simulink model "pada_plant_model_testing"  (R2022b)
settings: Solver=VariableStepAuto  StartTime=0.0  StopTime=20  RelTol=1e-3
values from neighbouring files (symbols this model uses):
  A_lon = [du_u,  du_w,   du_q,   du_theta ... (first row only)    [pada_linear_model.m]
  B_lon = [du_de,     du_dt ... (first row only)    [pada_linear_model.m]
  C_D0 = 0.0159    [pada_aero_coefficients.m]
  C_Dalpha = 0    [pada_aero_coefficients.m]
  C_Dde = 0    [pada_aero_coefficients.m]
  C_Dq = 0    [pada_aero_coefficients.m]
  C_l0 = 0.0033    [pada_aero_coefficients.m]
  C_L0 = 0.0193    [pada_aero_coefficients.m]
  C_Lalpha = 0.056    [pada_aero_coefficients.m]
  C_lbeta = -0.04415    [pada_aero_coefficients.m]
  C_lda = 0.0025326    [pada_aero_coefficients.m]
  C_Lde = 0    [pada_aero_coefficients.m]
  C_lon = eye(4)    [pada_linear_model.m]
  C_Lq = 3.48391    [pada_aero_coefficients.m]
  C_m0 = 0.00045    [pada_aero_coefficients.m]
  C_malpha = -0.3787    [pada_aero_coefficients.m]
  C_mde = 0    [pada_aero_coefficients.m]
  C_mq = -1.26832    [pada_aero_coefficients.m]
  C_n0 = 0    [pada_aero_coefficients.m]
  C_nbeta = 0.12637    [pada_aero_coefficients.m]
  C_nda = 0    [pada_aero_coefficients.m]
  C_Xde = C_Xde    [pada_linear_model.m]
  C_Y0 = 0    [pada_aero_coefficients.m]
  C_Ybeta = -0.6377    [pada_aero_coefficients.m]
  C_Yda = 0    [pada_aero_coefficients.m]
  C_Yp = -0.06787    [pada_aero_coefficients.m]
  C_Yr = 0.51996    [pada_aero_coefficients.m]
  C_Zde = C_Zde    [pada_linear_model.m]
  D_lon = zeros(4,2)    [pada_linear_model.m]
  g = 9.81    [pada_plant.m]
  J_x = 1    [pada_plant.m]
  J_xz = 1    [pada_plant.m]
  J_y = 1    [pada_plant.m]
  J_z = 1    [pada_plant.m]
  k_motor = 1    [pada_plant.m]
  m = 1    [pada_plant.m]
  q_0 = 0    [pada_linear_model.m]
  Ref_area = 1    [pada_plant.m]
  Ref_chord = 1    [pada_plant.m]
  Ref_span = 1    [pada_plant.m]
  rho = 1    [pada_plant.m]
  S_prop = 1    [pada_plant.m]
  theta_0 = 0.01    [pada_linear_model.m]
  u_0 = 10.0    (= 10)    [pada_linear_model.m]
  w_0 = 1.0    (= 1)    [pada_linear_model.m]
undefined symbols (not defined in the file or in its folder): C_Xda, C_Zda, K_lon
libraries: simulink_extras x5, slpidlib x4, shared6dof x3, aerolibasang x3, sharedtransform x1, uavutilslib x1
(part 1 of 2)
settings Model: Creator=zachary  LastModifiedBy=zacha

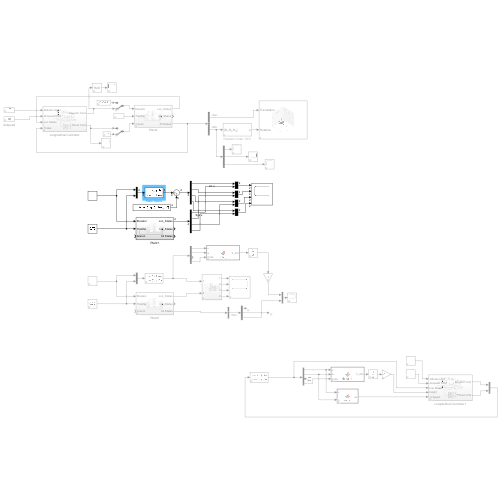
[thumbnail: Simulink's stored preview of the top-level diagram]
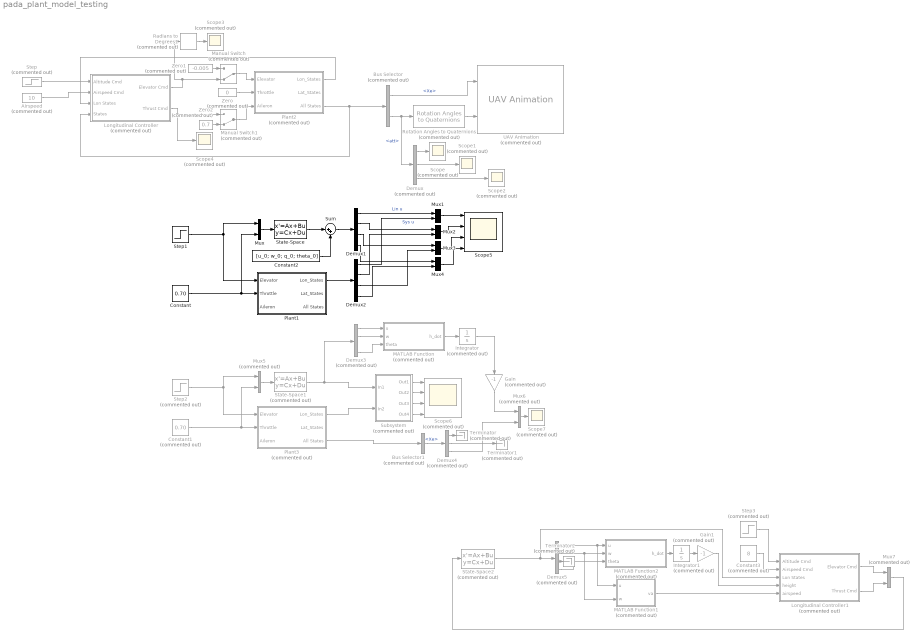
== system pada_plant_model_testing ==
  Airspeed : Constant  Commented=on  Value=10
  Bus Selector : BusSelector  Commented=on  OutputSignals=Xe,att
  Bus Selector1 : BusSelector  Commented=on  OutputSignals=Xe
  Constant : Constant  Value=0.70
  Constant1 : Constant  Commented=on  Value=0.70
  Constant2 : Constant  Value=[u_0; w_0; q_0; theta_0]
  Constant3 : Constant  Commented=on  Value=8
  Demux : Demux  Commented=on  Outputs=3
  Demux1 : Demux
  Demux2 : Demux
  Demux3 : Demux  Commented=on
  Demux4 : Demux  Commented=on  Outputs=3
  Demux5 : Demux  Commented=on
  Gain : Gain  Commented=on  Gain=-1
  Gain1 : Gain  Commented=on  Gain=-1
  Integrator : Integrator  Commented=on
  Integrator1 : Integrator  Commented=on
  Longitudinal Controller : Subsystem  Commented=on
  Longitudinal Controller1 : Subsystem  Commented=on
  MATLAB Function : MATLAB Function  Commented=on  TreatAsAtomicUnit=on
  MATLAB Function1 : MATLAB Function  Commented=on  TreatAsAtomicUnit=on
  MATLAB Function2 : MATLAB Function  Commented=on  TreatAsAtomicUnit=on
  Manual Switch : ManualSwitch  Commented=on  CurrentSetting=0
  Manual Switch1 : ManualSwitch  Commented=on  CurrentSetting=0
  Mux{,1..4} (5 alike) : Mux  Inputs=2
  Mux5 : Mux  Commented=on  Inputs=2
  Mux6 : Mux  Commented=on  Inputs=2
  Mux7 : Mux  Commented=on  Inputs=2
  Plant1 : Subsystem
  Plant2 : Subsystem  Commented=on
  Plant3 : Subsystem  Commented=on
  Radians to Degrees1 : simulink_extras/Transformations/Radians to Degrees  Commented=on
  Rotation Angles to Quaternions : sharedtransform/Rotation Angles to Quaternions  Commented=on  rotationOrder=ZYX  aMode=aMode
  Scope{,1..4,7} (6 alike) : Scope  Commented=on
  Scope5 : Scope  NumInputPorts=4
  Scope6 : Scope  Commented=on  NumInputPorts=4
  State-Space : StateSpace  A=A_lon  B=B_lon  C=C_lon  D=D_lon  InitialCondition=0
  State-Space1 : StateSpace  Commented=on  A=A_lon  B=B_lon  C=C_lon  D=D_lon  InitialCondition=0
  State-Space2 : StateSpace  Commented=on  A=A_lon  B=B_lon  C=C_lon  D=D_lon  InitialCondition=0
  Step : Step  Commented=on  After=0  SampleTime=0
  Step1 : Step  After=0.1  SampleTime=0
  Step2 : Step  Commented=on  After=0.1  SampleTime=0
  Step3 : Step  Commented=on  After=20  SampleTime=0
  Subsystem : Subsystem  Commented=on
  Sum : Sum  Inputs=|++
  Terminator : Terminator  Commented=on
  Terminator1 : Terminator  Commented=on
  Terminator2 : Terminator  Commented=on
  UAV Animation : uavutilslib/UAV Animation  Commented=on  UAVType=FixedWing  UAVSize=1  InertialZDirection=Down  SampleTime=-1
  Zero : Constant  Commented=on  Value=0  OutDataTypeStr=Inherit: Inherit via back propagation
  Zero1 : Constant  Commented=on  Value=-0.005  OutDataTypeStr=Inherit: Inherit via back propagation
  Zero2 : Constant  Commented=on  Value=0.7  OutDataTypeStr=Inherit: Inherit via back propagation
  wires:
  Plant2/3(All States) -> Bus Selector/1, Longitudinal Controller/4(States)
  Bus Selector/1 -> UAV Animation/1  "<Xe>"
  Bus Selector/2 -> Demux/1, Rotation Angles to Quaternions/1  "<att>"
  Rotation Angles to Quaternions/1 -> UAV Animation/2
  Zero/1 -> Plant2/2(Throttle)
  Zero2/1 -> Manual Switch1/2
  Zero1/1 -> Manual Switch/1
  Demux/1 -> Scope/1
  Demux/2 -> Scope1/1
  Demux/3 -> Scope2/1
  Manual Switch/1 -> Plant2/1(Elevator)
  Manual Switch1/1 -> Plant2/3(Aileron)
  Radians to Degrees1/1 -> Scope3/1
  Longitudinal Controller/1(Elevator Cmd) -> Radians to Degrees1/1, Manual Switch/2
  Longitudinal Controller/2(Thrust Cmd) -> Scope4/1, Manual Switch1/1
  Step/1 -> Longitudinal Controller/1(Altitude Cmd)
  Plant2/1(Lon_States) -> Longitudinal Controller/3(Lon States)
  Airspeed/1 -> Longitudinal Controller/2(Airspeed Cmd)
  Mux/1 -> State-Space/1
  State-Space/1 -> Sum/1
  Plant1/1(Lon_States) -> Demux2/1
  Step1/1 -> Mux/1, Plant1/1(Elevator)
  Constant/1 -> Mux/2, Plant1/2(Throttle)
  Mux1/1 -> Scope5/1
  Demux1/1 -> Mux1/1  "Lin u"
  Demux2/1 -> Mux1/2  "Sys u"
  Mux2/1 -> Scope5/2
  Mux3/1 -> Scope5/3
  Mux4/1 -> Scope5/4
  Demux1/2 -> Mux2/1
  Demux2/2 -> Mux2/2
  Demux1/3 -> Mux3/1
  Demux2/3 -> Mux3/2
  Demux1/4 -> Mux4/1
  Demux2/4 -> Mux4/2
  Constant1/1 -> Plant3/2(Throttle), Mux5/2
  Step2/1 -> Mux5/1, Plant3/1(Elevator)
  Mux5/1 -> State-Space1/1
  State-Space1/1 -> Demux3/1, Subsystem/1(In1)
  Plant3/1(Lon_States) -> Subsystem/2(In2)
  Subsystem/1(Out1) -> Scope6/1
  Subsystem/2(Out2) -> Scope6/2
  Subsystem/3(Out3) -> Scope6/3
  Subsystem/4(Out4) -> Scope6/4
  Demux3/1 -> MATLAB Function/1(u)
  Demux3/2 -> MATLAB Function/2(w)
  Demux3/4 -> MATLAB Function/3(theta)
  Plant3/3(All States) -> Bus Selector1/1
  Bus Selector1/1 -> Demux4/1  "<Xe>"
  MATLAB Function/1(h_dot) -> Integrator/1
  Mux6/1 -> Scope7/1
  Integrator/1 -> Gain/1
  Demux4/3 -> Mux6/2
  Demux4/1 -> Terminator/1
  Demux4/2 -> Terminator1/1
  Gain/1 -> Mux6/1
  Gain1/1 -> Longitudinal Controller1/4(height)
  Demux5/4 -> MATLAB Function2/3(theta)
  Demux5/2 -> MATLAB Function1/2(w), MATLAB Function2/2(w)
  State-Space2/1 -> Demux5/1, Longitudinal Controller1/3(Lon States)
  MATLAB Function2/1(h_dot) -> Integrator1/1
  Demux5/1 -> MATLAB Function1/1(u), MATLAB Function2/1(u)
  Integrator1/1 -> Gain1/1
  Demux5/3 -> Terminator2/1
  MATLAB Function1/1(va) -> Longitudinal Controller1/5(airspeed)
  Longitudinal Controller1/1(Elevator Cmd) -> Mux7/1
  Longitudinal Controller1/2(Thrust Cmd) -> Mux7/2
  Mux7/1 -> State-Space2/1
  Step3/1 -> Longitudinal Controller1/1(Altitude Cmd)
  Constant3/1 -> Longitudinal Controller1/2(Airspeed Cmd)
  Sum/1 -> Demux1/1
  Constant2/1 -> Sum/2

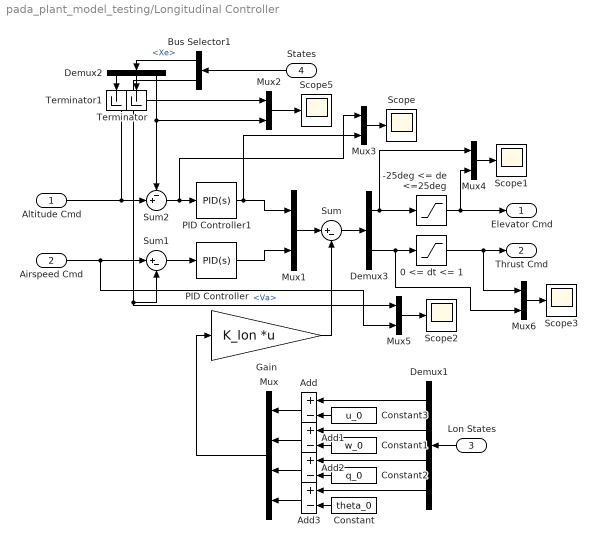
== system pada_plant_model_testing/Longitudinal Controller ==
  Altitude Cmd : Inport
  Airspeed Cmd : Inport  Port=2
  Lon States : Inport  Port=3
  States : Inport  Port=4
  -25deg <= de <=25deg : Saturate
  0 <= dt <= 1 : Saturate  UpperLimit=1  LowerLimit=0
  Add{,1..3} (4 alike) : Sum  Inputs=+-
  Bus Selector1 : BusSelector  OutputSignals=Xe,Va
  Constant : Constant  Value=theta_0  VectorParams1D=off
  Constant1 : Constant  Value=w_0  VectorParams1D=off
  Constant2 : Constant  Value=q_0  VectorParams1D=off
  Constant3 : Constant  Value=u_0  VectorParams1D=off
  Demux1 : Demux
  Demux2 : Demux  Outputs=3
  Demux3 : Demux  Outputs=2
  Gain : Gain  Gain=K_lon  Multiplication=Matrix(K*u)
  Mux : Mux
  Mux{1..6} (6 alike) : Mux  Inputs=2
  PID Controller : slpidlib/PID Controller  Controller=PID  Form=Parallel  TimeDomain=Continuous-time  UseExternalTs=off  SampleTime=-1  IntegratorMethod=Forward Euler  FilterMethod=Forward Euler  ControllerParametersSource=internal  P=0  I=0  UseKiTs=off  D=0  N=15  UseFilter=on  TunerSelectOption=Transfer Function Based (PID Tuner App)  InitialConditionSource=internal  InitialConditionForIntegrator=0  InitialConditionForFilter=0  DifferentiatorICPrevScaledInput=0  ExternalReset=none  TrackingMode=off  Kt=1  LimitOutput=off  SatLimitsSource=internal  UpperSaturationLimit=inf  LowerSaturationLimit=-inf  LinearizeAsGain=on  AntiWindupMode=none  Kb=1  LimitIntegrator=off  UpperIntegratorSaturationLimit=inf  LowerIntegratorSaturationLimit=-inf  POutMin=[]  POutMax=[]  IOutMin=[]  IOutMax=[]  DOutMin=[]  DOutMax=[]  NOutMin=[]  NOutMax=[]  SumOutMin=[]  SumOutMax=[]  SaturationOutMin=[]  SaturationOutMax=[]  PParamMin=[]  PParamMax=[]  IParamMin=[]  IParamMax=[]  DParamMin=[]  DParamMax=[]  NParamMin=[]  NParamMax=[]  KbParamMin=[]  KbParamMax=[]  KtParamMin=[]  KtParamMax=[]  KbOutMin=[]  KbOutMax=[]  KtOutMin=[]  KtOutMax=[]  IntegratorOutMin=[]  IntegratorOutMax=[]  FilterOutMin=[]  FilterOutMax=[]  SumI1OutMin=[]  SumI1OutMax=[]  SumI2OutMin=[]  SumI2OutMax=[]  SumI3OutMin=[]  SumI3OutMax=[]  SumI4OutMin=[]  SumI4OutMax=[]  SumDOutMin=[]  SumDOutMax=[]  DifferentiatorOutMin=[]  DifferentiatorOutMax=[]  FilterDiffOutCoefMin=[]  FilterDiffOutCoefMax=[]  ReciprocalOutMin=[]  ReciprocalOutMax=[]  SumDenOutMin=[]  SumDenOutMax=[]  SumNumOutMin=[]  SumNumOutMax=[]  DivideOutMin=[]  DivideOutMax=[]  UdiffTsProdOutMin=[]  UdiffTsProdOutMax=[]  NTsProdOutMin=[]  NTsProdOutMax=[]  UintegralTsProdOutMin=[]  UintegralTsProdOutMax=[]  UngainTsProdOutMin=[]  UngainTsProdOutMax=[]  ClampingZeroOutDataTypeStr=Inherit: Inherit via back propagation  ClampingZeroOutMin=[]  ClampingZeroOutMax=[]  FilterDenConstantOutDataTypeStr=Inherit: Inherit via back propagation  FilterDenConstantOutMin=[]  FilterDenConstantOutMax=[]  PCopyOutDataTypeStr=Inherit: Inherit via back propagation  PCopyOutMin=[]  PCopyOutMax=[]  NCopyOutDataTypeStr=Inherit: Inherit via back propagation  NCopyOutMin=[]  NCopyOutMax=[]  IntegratorContinuousStateAttributes=''  IntegratorStateMustResolveToSignalObject=off  IntegratorRTWStateStorageClass=Auto  FilterContinuousStateAttributes=''  FilterStateMustResolveToSignalObject=off  FilterRTWStateStorageClass=Auto  ParallelPVariant=InternalParameters  IdealPVariant=Disabled  IVariant=InternalParameters  DVariant=InternalParameters  IntegratorVariant=Continuous  SatVariant=Disabled  AWVariant=Passthrough  PCopyVariant=Disabled  TRVariant=Disabled  FdbkBlocksVariant=Forward  IdealPFdbkVariant=Disabled  SatFdbkVariant=Disabled  DerivativeFilterVariant=ContFilter  NVariant=InternalParameters  NCopyVariant=Disabled  FilterICVariant=InternalICsFilter  IntegratorICVariant=InternalICs  ExternalResetVariant=Disabled  TRSumVariant=Passthrough  SumFdbkVariant=Disabled  SumVariant=Sum_PID  TsampFilterVariant=InternalTs  TsampNgainVariant=Passthrough  TsampIntegralVariant=Passthrough  ExternalSaturationOutDataTypeStr=Inherit: Same as second input
  PID Controller1 : slpidlib/PID Controller  Controller=PID  Form=Parallel  TimeDomain=Continuous-time  UseExternalTs=off  SampleTime=-1  IntegratorMethod=Forward Euler  FilterMethod=Forward Euler  ControllerParametersSource=internal  P=1  I=0  UseKiTs=off  D=0  N=15  UseFilter=on  TunerSelectOption=Transfer Function Based (PID Tuner App)  InitialConditionSource=internal  InitialConditionForIntegrator=0  InitialConditionForFilter=0  DifferentiatorICPrevScaledInput=0  ExternalReset=none  TrackingMode=off  Kt=1  LimitOutput=off  SatLimitsSource=internal  UpperSaturationLimit=inf  LowerSaturationLimit=-inf  LinearizeAsGain=on  AntiWindupMode=none  Kb=1  LimitIntegrator=off  UpperIntegratorSaturationLimit=inf  LowerIntegratorSaturationLimit=-inf  POutMin=[]  POutMax=[]  IOutMin=[]  IOutMax=[]  DOutMin=[]  DOutMax=[]  NOutMin=[]  NOutMax=[]  SumOutMin=[]  SumOutMax=[]  SaturationOutMin=[]  SaturationOutMax=[]  PParamMin=[]  PParamMax=[]  IParamMin=[]  IParamMax=[]  DParamMin=[]  DParamMax=[]  NParamMin=[]  NParamMax=[]  KbParamMin=[]  KbParamMax=[]  KtParamMin=[]  KtParamMax=[]  KbOutMin=[]  KbOutMax=[]  KtOutMin=[]  KtOutMax=[]  IntegratorOutMin=[]  IntegratorOutMax=[]  FilterOutMin=[]  FilterOutMax=[]  SumI1OutMin=[]  SumI1OutMax=[]  SumI2OutMin=[]  SumI2OutMax=[]  SumI3OutMin=[]  SumI3OutMax=[]  SumI4OutMin=[]  SumI4OutMax=[]  SumDOutMin=[]  SumDOutMax=[]  DifferentiatorOutMin=[]  DifferentiatorOutMax=[]  FilterDiffOutCoefMin=[]  FilterDiffOutCoefMax=[]  ReciprocalOutMin=[]  ReciprocalOutMax=[]  SumDenOutMin=[]  SumDenOutMax=[]  SumNumOutMin=[]  SumNumOutMax=[]  DivideOutMin=[]  DivideOutMax=[]  UdiffTsProdOutMin=[]  UdiffTsProdOutMax=[]  NTsProdOutMin=[]  NTsProdOutMax=[]  UintegralTsProdOutMin=[]  UintegralTsProdOutMax=[]  UngainTsProdOutMin=[]  UngainTsProdOutMax=[]  ClampingZeroOutDataTypeStr=Inherit: Inherit via back propagation  ClampingZeroOutMin=[]  ClampingZeroOutMax=[]  FilterDenConstantOutDataTypeStr=Inherit: Inherit via back propagation  FilterDenConstantOutMin=[]  FilterDenConstantOutMax=[]  PCopyOutDataTypeStr=Inherit: Inherit via back propagation  PCopyOutMin=[]  PCopyOutMax=[]  NCopyOutDataTypeStr=Inherit: Inherit via back propagation  NCopyOutMin=[]  NCopyOutMax=[]  IntegratorContinuousStateAttributes=''  IntegratorStateMustResolveToSignalObject=off  IntegratorRTWStateStorageClass=Auto  FilterContinuousStateAttributes=''  FilterStateMustResolveToSignalObject=off  FilterRTWStateStorageClass=Auto  ParallelPVariant=InternalParameters  IdealPVariant=Disabled  IVariant=InternalParameters  DVariant=InternalParameters  IntegratorVariant=Continuous  SatVariant=Disabled  AWVariant=Passthrough  PCopyVariant=Disabled  TRVariant=Disabled  FdbkBlocksVariant=Forward  IdealPFdbkVariant=Disabled  SatFdbkVariant=Disabled  DerivativeFilterVariant=ContFilter  NVariant=InternalParameters  NCopyVariant=Disabled  FilterICVariant=InternalICsFilter  IntegratorICVariant=InternalICs  ExternalResetVariant=Disabled  TRSumVariant=Passthrough  SumFdbkVariant=Disabled  SumVariant=Sum_PID  TsampFilterVariant=InternalTs  TsampNgainVariant=Passthrough  TsampIntegralVariant=Passthrough  ExternalSaturationOutDataTypeStr=Inherit: Same as second input
  Scope{,1..3,5} (5 alike) : Scope
  Sum : Sum  Inputs=|+-
  Sum1 : Sum  Inputs=|+-
  Sum2 : Sum  Inputs=-+|
  Terminator : Terminator
  Terminator1 : Terminator
  Elevator Cmd : Outport
  Thrust Cmd : Outport  Port=2
  wires:
  Demux1/3 -> Add2/1
  Constant3/1 -> Add/2
  Mux1/1 -> Sum/1
  Bus Selector1/1 -> Demux2/1  "<Xe>"
  Demux1/2 -> Add1/1
  Demux3/1 -> Mux4/1, -25deg <= de <=25deg/1
  Mux/1 -> Gain/1
  PID Controller1/1 -> Mux3/2, Mux1/1
  Altitude Cmd/1 -> Mux2/1, Sum2/2
  Demux2/3 -> Sum2/1, Mux2/2
  Add3/1 -> Mux/4
  Mux2/1 -> Scope5/1
  Demux1/1 -> Add/1
  Constant/1 -> Add3/2
  States/1 -> Bus Selector1/1
  Demux3/2 -> Mux6/2, 0 <= dt <= 1/1
  Sum1/1 -> PID Controller/1
  Sum/1 -> Demux3/1
  Sum2/1 -> Mux3/1, PID Controller1/1
  PID Controller/1 -> Mux1/2
  0 <= dt <= 1/1 -> Mux6/1, Thrust Cmd/1
  Gain/1 -> Sum/2
  Add/1 -> Mux/1
  Constant1/1 -> Add1/2
  Add1/1 -> Mux/2
  -25deg <= de <=25deg/1 -> Mux4/2, Elevator Cmd/1
  Constant2/1 -> Add2/2
  Demux1/4 -> Add3/1
  Add2/1 -> Mux/3
  Bus Selector1/2 -> Mux5/1, Sum1/2  "<Va>"
  Airspeed Cmd/1 -> Mux5/2, Sum1/1
  Lon States/1 -> Demux1/1
  Demux2/2 -> Terminator/1
  Demux2/1 -> Terminator1/1
  Mux3/1 -> Scope/1
  Mux4/1 -> Scope1/1
  Mux5/1 -> Scope2/1
  Mux6/1 -> Scope3/1

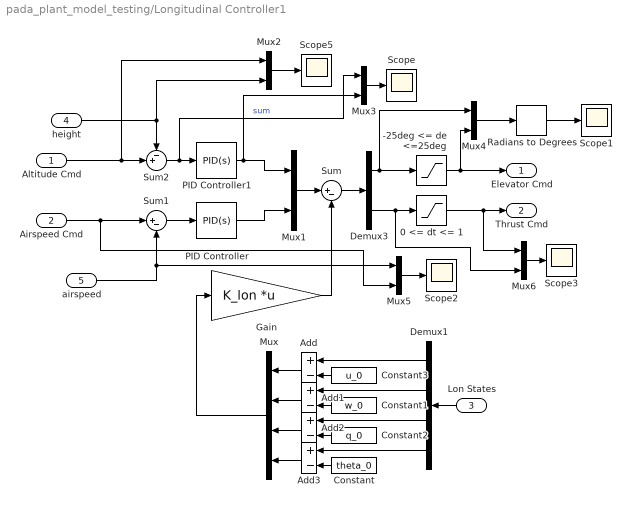
== system pada_plant_model_testing/Longitudinal Controller1 ==
  Altitude Cmd : Inport
  Airspeed Cmd : Inport  Port=2
  Lon States : Inport  Port=3
  height : Inport  Port=4
  airspeed : Inport  Port=5
  -25deg <= de <=25deg : Saturate
  0 <= dt <= 1 : Saturate  UpperLimit=1  LowerLimit=0
  Add{,1..3} (4 alike) : Sum  Inputs=+-
  Constant : Constant  Value=theta_0  VectorParams1D=off
  Constant1 : Constant  Value=w_0  VectorParams1D=off
  Constant2 : Constant  Value=q_0  VectorParams1D=off
  Constant3 : Constant  Value=u_0  VectorParams1D=off
  Demux1 : Demux
  Demux3 : Demux  Outputs=2
  Gain : Gain  Gain=K_lon  Multiplication=Matrix(K*u)
  Mux : Mux
  Mux{1..6} (6 alike) : Mux  Inputs=2
  PID Controller : slpidlib/PID Controller  Controller=PID  Form=Parallel  TimeDomain=Continuous-time  UseExternalTs=off  SampleTime=-1  IntegratorMethod=Forward Euler  FilterMethod=Forward Euler  ControllerParametersSource=internal  P=1  I=0  UseKiTs=off  D=0  N=15  UseFilter=on  TunerSelectOption=Transfer Function Based (PID Tuner App)  InitialConditionSource=internal  InitialConditionForIntegrator=0  InitialConditionForFilter=0  DifferentiatorICPrevScaledInput=0  ExternalReset=none  TrackingMode=off  Kt=1  LimitOutput=off  SatLimitsSource=internal  UpperSaturationLimit=inf  LowerSaturationLimit=-inf  LinearizeAsGain=on  AntiWindupMode=none  Kb=1  LimitIntegrator=off  UpperIntegratorSaturationLimit=inf  LowerIntegratorSaturationLimit=-inf  POutMin=[]  POutMax=[]  IOutMin=[]  IOutMax=[]  DOutMin=[]  DOutMax=[]  NOutMin=[]  NOutMax=[]  SumOutMin=[]  SumOutMax=[]  SaturationOutMin=[]  SaturationOutMax=[]  PParamMin=[]  PParamMax=[]  IParamMin=[]  IParamMax=[]  DParamMin=[]  DParamMax=[]  NParamMin=[]  NParamMax=[]  KbParamMin=[]  KbParamMax=[]  KtParamMin=[]  KtParamMax=[]  KbOutMin=[]  KbOutMax=[]  KtOutMin=[]  KtOutMax=[]  IntegratorOutMin=[]  IntegratorOutMax=[]  FilterOutMin=[]  FilterOutMax=[]  SumI1OutMin=[]  SumI1OutMax=[]  SumI2OutMin=[]  SumI2OutMax=[]  SumI3OutMin=[]  SumI3OutMax=[]  SumI4OutMin=[]  SumI4OutMax=[]  SumDOutMin=[]  SumDOutMax=[]  DifferentiatorOutMin=[]  DifferentiatorOutMax=[]  FilterDiffOutCoefMin=[]  FilterDiffOutCoefMax=[]  ReciprocalOutMin=[]  ReciprocalOutMax=[]  SumDenOutMin=[]  SumDenOutMax=[]  SumNumOutMin=[]  SumNumOutMax=[]  DivideOutMin=[]  DivideOutMax=[]  UdiffTsProdOutMin=[]  UdiffTsProdOutMax=[]  NTsProdOutMin=[]  NTsProdOutMax=[]  UintegralTsProdOutMin=[]  UintegralTsProdOutMax=[]  UngainTsProdOutMin=[]  UngainTsProdOutMax=[]  ClampingZeroOutDataTypeStr=Inherit: Inherit via back propagation  ClampingZeroOutMin=[]  ClampingZeroOutMax=[]  FilterDenConstantOutDataTypeStr=Inherit: Inherit via back propagation  FilterDenConstantOutMin=[]  FilterDenConstantOutMax=[]  PCopyOutDataTypeStr=Inherit: Inherit via back propagation  PCopyOutMin=[]  PCopyOutMax=[]  NCopyOutDataTypeStr=Inherit: Inherit via back propagation  NCopyOutMin=[]  NCopyOutMax=[]  IntegratorContinuousStateAttributes=''  IntegratorStateMustResolveToSignalObject=off  IntegratorRTWStateStorageClass=Auto  FilterContinuousStateAttributes=''  FilterStateMustResolveToSignalObject=off  FilterRTWStateStorageClass=Auto  ParallelPVariant=InternalParameters  IdealPVariant=Disabled  IVariant=InternalParameters  DVariant=InternalParameters  IntegratorVariant=Continuous  SatVariant=Disabled  AWVariant=Passthrough  PCopyVariant=Disabled  TRVariant=Disabled  FdbkBlocksVariant=Forward  IdealPFdbkVariant=Disabled  SatFdbkVariant=Disabled  DerivativeFilterVariant=ContFilter  NVariant=InternalParameters  NCopyVariant=Disabled  FilterICVariant=InternalICsFilter  IntegratorICVariant=InternalICs  ExternalResetVariant=Disabled  TRSumVariant=Passthrough  SumFdbkVariant=Disabled  SumVariant=Sum_PID  TsampFilterVariant=InternalTs  TsampNgainVariant=Passthrough  TsampIntegralVariant=Passthrough  ExternalSaturationOutDataTypeStr=Inherit: Same as second input
  PID Controller1 : slpidlib/PID Controller  Controller=PID  Form=Parallel  TimeDomain=Continuous-time  UseExternalTs=off  SampleTime=-1  IntegratorMethod=Forward Euler  FilterMethod=Forward Euler  ControllerParametersSource=internal  P=1  I=0.1  UseKiTs=off  D=0.1  N=15  UseFilter=on  TunerSelectOption=Transfer Function Based (PID Tuner App)  InitialConditionSource=internal  InitialConditionForIntegrator=0  InitialConditionForFilter=0  DifferentiatorICPrevScaledInput=0  ExternalReset=none  TrackingMode=off  Kt=1  LimitOutput=off  SatLimitsSource=internal  UpperSaturationLimit=inf  LowerSaturationLimit=-inf  LinearizeAsGain=on  AntiWindupMode=none  Kb=1  LimitIntegrator=off  UpperIntegratorSaturationLimit=inf  LowerIntegratorSaturationLimit=-inf  POutMin=[]  POutMax=[]  IOutMin=[]  IOutMax=[]  DOutMin=[]  DOutMax=[]  NOutMin=[]  NOutMax=[]  SumOutMin=[]  SumOutMax=[]  SaturationOutMin=[]  SaturationOutMax=[]  PParamMin=[]  PParamMax=[]  IParamMin=[]  IParamMax=[]  DParamMin=[]  DParamMax=[]  NParamMin=[]  NParamMax=[]  KbParamMin=[]  KbParamMax=[]  KtParamMin=[]  KtParamMax=[]  KbOutMin=[]  KbOutMax=[]  KtOutMin=[]  KtOutMax=[]  IntegratorOutMin=[]  IntegratorOutMax=[]  FilterOutMin=[]  FilterOutMax=[]  SumI1OutMin=[]  SumI1OutMax=[]  SumI2OutMin=[]  SumI2OutMax=[]  SumI3OutMin=[]  SumI3OutMax=[]  SumI4OutMin=[]  SumI4OutMax=[]  SumDOutMin=[]  SumDOutMax=[]  DifferentiatorOutMin=[]  DifferentiatorOutMax=[]  FilterDiffOutCoefMin=[]  FilterDiffOutCoefMax=[]  ReciprocalOutMin=[]  ReciprocalOutMax=[]  SumDenOutMin=[]  SumDenOutMax=[]  SumNumOutMin=[]  SumNumOutMax=[]  DivideOutMin=[]  DivideOutMax=[]  UdiffTsProdOutMin=[]  UdiffTsProdOutMax=[]  NTsProdOutMin=[]  NTsProdOutMax=[]  UintegralTsProdOutMin=[]  UintegralTsProdOutMax=[]  UngainTsProdOutMin=[]  UngainTsProdOutMax=[]  ClampingZeroOutDataTypeStr=Inherit: Inherit via back propagation  ClampingZeroOutMin=[]  ClampingZeroOutMax=[]  FilterDenConstantOutDataTypeStr=Inherit: Inherit via back propagation  FilterDenConstantOutMin=[]  FilterDenConstantOutMax=[]  PCopyOutDataTypeStr=Inherit: Inherit via back propagation  PCopyOutMin=[]  PCopyOutMax=[]  NCopyOutDataTypeStr=Inherit: Inherit via back propagation  NCopyOutMin=[]  NCopyOutMax=[]  IntegratorContinuousStateAttributes=''  IntegratorStateMustResolveToSignalObject=off  IntegratorRTWStateStorageClass=Auto  FilterContinuousStateAttributes=''  FilterStateMustResolveToSignalObject=off  FilterRTWStateStorageClass=Auto  ParallelPVariant=InternalParameters  IdealPVariant=Disabled  IVariant=InternalParameters  DVariant=InternalParameters  IntegratorVariant=Continuous  SatVariant=Disabled  AWVariant=Passthrough  PCopyVariant=Disabled  TRVariant=Disabled  FdbkBlocksVariant=Forward  IdealPFdbkVariant=Disabled  SatFdbkVariant=Disabled  DerivativeFilterVariant=ContFilter  NVariant=InternalParameters  NCopyVariant=Disabled  FilterICVariant=InternalICsFilter  IntegratorICVariant=InternalICs  ExternalResetVariant=Disabled  TRSumVariant=Passthrough  SumFdbkVariant=Disabled  SumVariant=Sum_PID  TsampFilterVariant=InternalTs  TsampNgainVariant=Passthrough  TsampIntegralVariant=Passthrough  ExternalSaturationOutDataTypeStr=Inherit: Same as second input
  Radians to Degrees : simulink_extras/Transformations/Radians to Degrees
  Scope{,1..3,5} (5 alike) : Scope
  Sum : Sum  Inputs=|+-
  Sum1 : Sum  Inputs=|+-
  Sum2 : Sum  Inputs=-+|
  Elevator Cmd : Outport
  Thrust Cmd : Outport  Port=2
  wires:
  Demux1/3 -> Add2/1
  Constant3/1 -> Add/2
  Mux1/1 -> Sum/1
  Demux1/2 -> Add1/1
  Demux3/1 -> Mux4/1, -25deg <= de <=25deg/1
  Mux/1 -> Gain/1
  PID Controller1/1 -> Mux3/2, Mux1/1
  Altitude Cmd/1 -> Mux2/1, Sum2/2
  Add3/1 -> Mux/4
  Mux2/1 -> Scope5/1
  Demux1/1 -> Add/1
  Constant/1 -> Add3/2
  Demux3/2 -> Mux6/2, 0 <= dt <= 1/1
  Sum1/1 -> PID Controller/1
  Sum/1 -> Demux3/1
  Sum2/1 -> Mux3/1, PID Controller1/1  "sum"
  PID Controller/1 -> Mux1/2
  0 <= dt <= 1/1 -> Mux6/1, Thrust Cmd/1
  Gain/1 -> Sum/2
  Add/1 -> Mux/1
  Constant1/1 -> Add1/2
  Add1/1 -> Mux/2
  -25deg <= de <=25deg/1 -> Mux4/2, Elevator Cmd/1
  Constant2/1 -> Add2/2
  Demux1/4 -> Add3/1
  Add2/1 -> Mux/3
  Airspeed Cmd/1 -> Mux5/2, Sum1/1
  Lon States/1 -> Demux1/1
  Mux3/1 -> Scope/1
  Mux4/1 -> Radians to Degrees/1
  Mux5/1 -> Scope2/1
  Mux6/1 -> Scope3/1
  airspeed/1 -> Mux5/1, Sum1/2
  height/1 -> Mux2/2, Sum2/1
  Radians to Degrees/1 -> Scope1/1

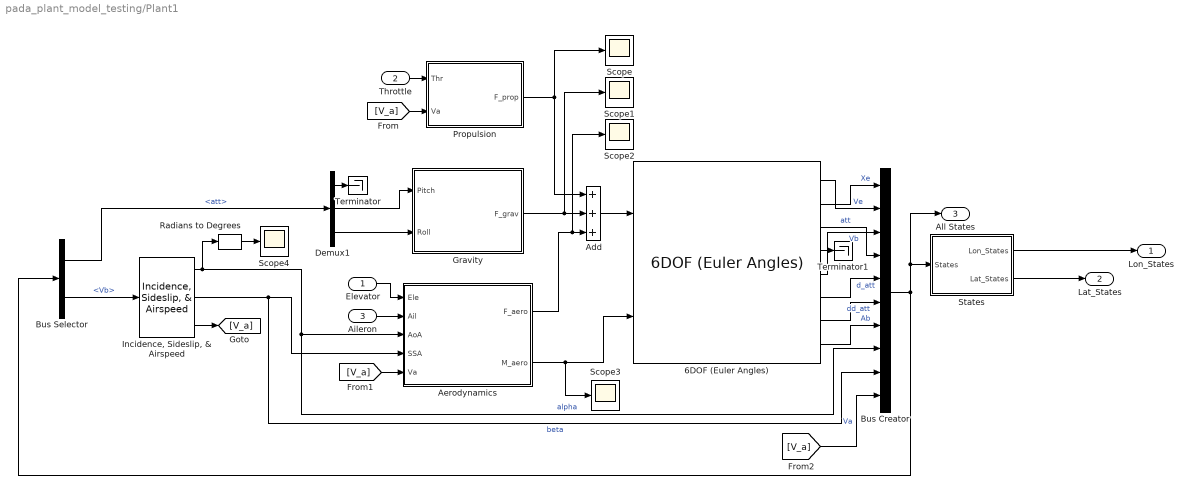
== system pada_plant_model_testing/Plant1 ==
  Elevator : Inport
  Throttle : Inport  Port=2
  Aileron : Inport  Port=3
  6DOF (Euler Angles) : shared6dof/6DOF (Euler Angles)  units=Metric (MKS)  mtype=Fixed  rep=Euler Angles  xme_0=[0 0 0]  Vm_0=[u_0 0 w_0]  eul_0=[0 0 0]  pm_0=[0 0 0]  mass_0=m  mass_e=0.5  mass_f=2.0  inertia=[J_x, 0, -J_xz; 0, J_y, 0; -J_xz, 0, J_z]  inertia_e=eye(3)  inertia_f=2*eye(3)  k_quat=1.0  vre_flag=on  abi_flag=off  aMode=0  xme_statename=''  Vm_statename=''  eul_statename=''  quat_statename=''  pm_statename=''  mass_statename=''
  Add : Sum  Inputs=+++
  Aerodynamics : Subsystem
  Bus Creator : BusCreator  Inputs=10
  Bus Selector : BusSelector  OutputSignals=att,Vb
  Demux1 : Demux  Outputs=3
  Gravity : Subsystem
  "Incidence, Sideslip, & Airspeed" : aerolibasang/Incidence, Sideslip, & Airspeed
  Propulsion : Subsystem
  Radians to Degrees : simulink_extras/Transformations/Radians to Degrees
  Scope{,1..4} (5 alike) : Scope
  States : Subsystem
  Terminator : Terminator
  Terminator1 : Terminator
  Lon_States : Outport
  Lat_States : Outport  Port=2
  All States : Outport  Port=3
  wires:
  Bus Creator/1 -> All States/1, States/1(States), Bus Selector/1
  Add/1 -> 6DOF (Euler Angles)/1
  Gravity/1(F_grav) -> Add/2, Scope1/1
  Propulsion/1(F_prop) -> Add/1, Scope/1
  "Incidence, Sideslip, & Airspeed"/2 -> Bus Creator/9, Aerodynamics/4(SSA)  "beta"
  Aerodynamics/2(M_aero) -> Scope3/1, 6DOF (Euler Angles)/2
  "Incidence, Sideslip, & Airspeed"/1 -> Bus Creator/8, Aerodynamics/3(AoA), Radians to Degrees/1  "alpha"
  Throttle/1 -> Propulsion/1(Thr)
  Elevator/1 -> Aerodynamics/1(Ele)
  6DOF (Euler Angles)/6 -> Bus Creator/5  "d_att"
  6DOF (Euler Angles)/4 -> Terminator1/1
  Aileron/1 -> Aerodynamics/2(Ail)
  Bus Selector/1 -> Demux1/1  "<att>"
  Demux1/1 -> Terminator/1
  6DOF (Euler Angles)/5 -> Bus Creator/3  "Vb"
  Demux1/2 -> Gravity/1(Pitch)
  6DOF (Euler Angles)/2 -> Bus Creator/1  "Xe"
  6DOF (Euler Angles)/7 -> Bus Creator/6  "dd_att"
  6DOF (Euler Angles)/8 -> Bus Creator/7  "Ab"
  6DOF (Euler Angles)/1 -> Bus Creator/2  "Ve"
  6DOF (Euler Angles)/3 -> Bus Creator/4  "att"
  Demux1/3 -> Gravity/2(Roll)
  Bus Selector/2 -> "Incidence, Sideslip, & Airspeed"/1  "<Vb>"
  States/2(Lat_States) -> Lat_States/1
  States/1(Lon_States) -> Lon_States/1
  [V_a] -> Propulsion/2(Va)
  [V_a] -> Aerodynamics/5(Va)
  "Incidence, Sideslip, & Airspeed"/3 -> [V_a]
  Aerodynamics/1(F_aero) -> Scope2/1, Add/3
  Radians to Degrees/1 -> Scope4/1
  [V_a] -> Bus Creator/10  "Va"

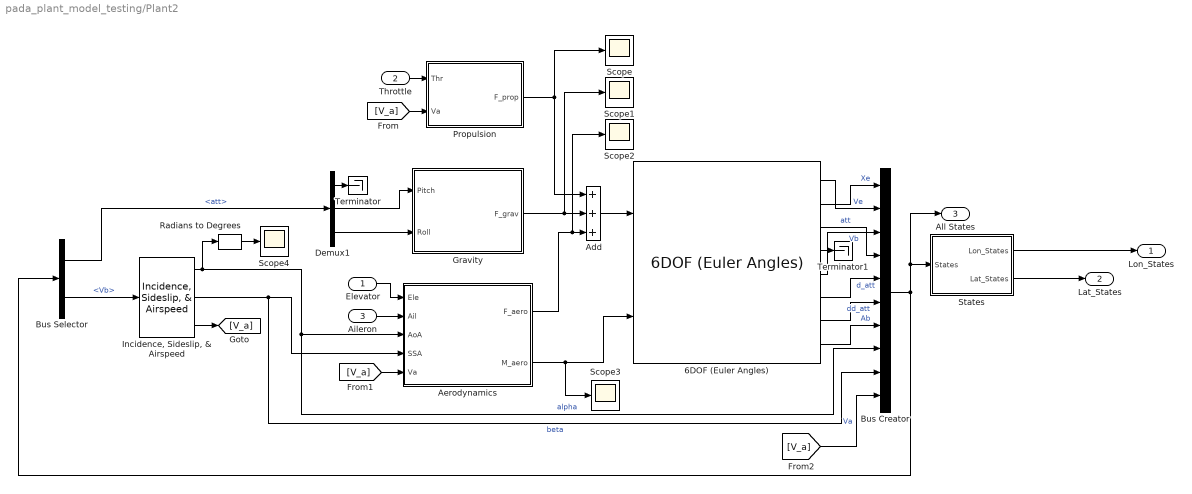
== system pada_plant_model_testing/Plant2 ==
  Elevator : Inport
  Throttle : Inport  Port=2
  Aileron : Inport  Port=3
  6DOF (Euler Angles) : shared6dof/6DOF (Euler Angles)  units=Metric (MKS)  mtype=Fixed  rep=Euler Angles  xme_0=[0 0 0]  Vm_0=[0 0 0]  eul_0=[0 0 0]  pm_0=[0 0 0]  mass_0=m  mass_e=0.5  mass_f=2.0  inertia=[J_x, 0, -J_xz; 0, J_y, 0; -J_xz, 0, J_z]  inertia_e=eye(3)  inertia_f=2*eye(3)  k_quat=1.0  vre_flag=on  abi_flag=off  aMode=0  xme_statename=''  Vm_statename=''  eul_statename=''  quat_statename=''  pm_statename=''  mass_statename=''
  Add : Sum  Inputs=+++
  Aerodynamics : Subsystem
  Bus Creator : BusCreator  Inputs=10
  Bus Selector : BusSelector  OutputSignals=att,Vb
  Demux1 : Demux  Outputs=3
  Gravity : Subsystem
  "Incidence, Sideslip, & Airspeed" : aerolibasang/Incidence, Sideslip, & Airspeed
  Propulsion : Subsystem
  Radians to Degrees : simulink_extras/Transformations/Radians to Degrees
  Scope{,1..4} (5 alike) : Scope
  States : Subsystem
  Terminator : Terminator
  Terminator1 : Terminator
  Lon_States : Outport
  Lat_States : Outport  Port=2
  All States : Outport  Port=3
  wires:
  Bus Creator/1 -> All States/1, States/1(States), Bus Selector/1
  Add/1 -> 6DOF (Euler Angles)/1
  Gravity/1(F_grav) -> Add/2, Scope1/1
  Propulsion/1(F_prop) -> Add/1, Scope/1
  "Incidence, Sideslip, & Airspeed"/2 -> Bus Creator/9, Aerodynamics/4(SSA)  "beta"
  Aerodynamics/2(M_aero) -> Scope3/1, 6DOF (Euler Angles)/2
  "Incidence, Sideslip, & Airspeed"/1 -> Bus Creator/8, Aerodynamics/3(AoA), Radians to Degrees/1  "alpha"
  Throttle/1 -> Propulsion/1(Thr)
  Elevator/1 -> Aerodynamics/1(Ele)
  6DOF (Euler Angles)/6 -> Bus Creator/5  "d_att"
  6DOF (Euler Angles)/4 -> Terminator1/1
  Aileron/1 -> Aerodynamics/2(Ail)
  Bus Selector/1 -> Demux1/1  "<att>"
  Demux1/1 -> Terminator/1
  6DOF (Euler Angles)/5 -> Bus Creator/3  "Vb"
  Demux1/2 -> Gravity/1(Pitch)
  6DOF (Euler Angles)/2 -> Bus Creator/1  "Xe"
  6DOF (Euler Angles)/7 -> Bus Creator/6  "dd_att"
  6DOF (Euler Angles)/8 -> Bus Creator/7  "Ab"
  6DOF (Euler Angles)/1 -> Bus Creator/2  "Ve"
  6DOF (Euler Angles)/3 -> Bus Creator/4  "att"
  Demux1/3 -> Gravity/2(Roll)
  Bus Selector/2 -> "Incidence, Sideslip, & Airspeed"/1  "<Vb>"
  States/2(Lat_States) -> Lat_States/1
  States/1(Lon_States) -> Lon_States/1
  [V_a] -> Propulsion/2(Va)
  [V_a] -> Aerodynamics/5(Va)
  "Incidence, Sideslip, & Airspeed"/3 -> [V_a]
  Aerodynamics/1(F_aero) -> Scope2/1, Add/3
  Radians to Degrees/1 -> Scope4/1
  [V_a] -> Bus Creator/10  "Va"

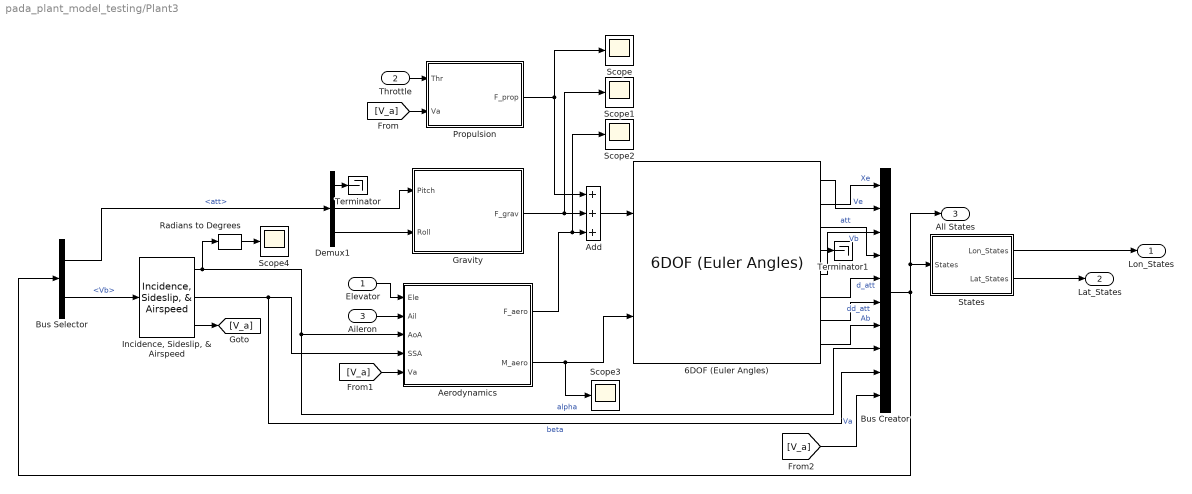
== system pada_plant_model_testing/Plant3 ==
  Elevator : Inport
  Throttle : Inport  Port=2
  Aileron : Inport  Port=3
  6DOF (Euler Angles) : shared6dof/6DOF (Euler Angles)  units=Metric (MKS)  mtype=Fixed  rep=Euler Angles  xme_0=[0 0 0]  Vm_0=[0 0 0]  eul_0=[0 0 0]  pm_0=[0 0 0]  mass_0=m  mass_e=0.5  mass_f=2.0  inertia=[J_x, 0, -J_xz; 0, J_y, 0; -J_xz, 0, J_z]  inertia_e=eye(3)  inertia_f=2*eye(3)  k_quat=1.0  vre_flag=on  abi_flag=off  aMode=0  xme_statename=''  Vm_statename=''  eul_statename=''  quat_statename=''  pm_statename=''  mass_statename=''
  Add : Sum  Inputs=+++
  Aerodynamics : Subsystem
  Bus Creator : BusCreator  Inputs=10
  Bus Selector : BusSelector  OutputSignals=att,Vb
  Demux1 : Demux  Outputs=3
  Gravity : Subsystem
  "Incidence, Sideslip, & Airspeed" : aerolibasang/Incidence, Sideslip, & Airspeed
  Propulsion : Subsystem
  Radians to Degrees : simulink_extras/Transformations/Radians to Degrees
  Scope{,1..4} (5 alike) : Scope
  States : Subsystem
  Terminator : Terminator
  Terminator1 : Terminator
  Lon_States : Outport
  Lat_States : Outport  Port=2
  All States : Outport  Port=3
  wires:
  Bus Creator/1 -> All States/1, States/1(States), Bus Selector/1
  Add/1 -> 6DOF (Euler Angles)/1
  Gravity/1(F_grav) -> Add/2, Scope1/1
  Propulsion/1(F_prop) -> Add/1, Scope/1
  "Incidence, Sideslip, & Airspeed"/2 -> Bus Creator/9, Aerodynamics/4(SSA)  "beta"
  Aerodynamics/2(M_aero) -> Scope3/1, 6DOF (Euler Angles)/2
  "Incidence, Sideslip, & Airspeed"/1 -> Bus Creator/8, Aerodynamics/3(AoA), Radians to Degrees/1  "alpha"
  Throttle/1 -> Propulsion/1(Thr)
  Elevator/1 -> Aerodynamics/1(Ele)
  6DOF (Euler Angles)/6 -> Bus Creator/5  "d_att"
  6DOF (Euler Angles)/4 -> Terminator1/1
  Aileron/1 -> Aerodynamics/2(Ail)
  Bus Selector/1 -> Demux1/1  "<att>"
  Demux1/1 -> Terminator/1
  6DOF (Euler Angles)/5 -> Bus Creator/3  "Vb"
  Demux1/2 -> Gravity/1(Pitch)
  6DOF (Euler Angles)/2 -> Bus Creator/1  "Xe"
  6DOF (Euler Angles)/7 -> Bus Creator/6  "dd_att"
  6DOF (Euler Angles)/8 -> Bus Creator/7  "Ab"
  6DOF (Euler Angles)/1 -> Bus Creator/2  "Ve"
  6DOF (Euler Angles)/3 -> Bus Creator/4  "att"
  Demux1/3 -> Gravity/2(Roll)
  Bus Selector/2 -> "Incidence, Sideslip, & Airspeed"/1  "<Vb>"
  States/2(Lat_States) -> Lat_States/1
  States/1(Lon_States) -> Lon_States/1
  [V_a] -> Propulsion/2(Va)
  [V_a] -> Aerodynamics/5(Va)
  "Incidence, Sideslip, & Airspeed"/3 -> [V_a]
  Aerodynamics/1(F_aero) -> Scope2/1, Add/3
  Radians to Degrees/1 -> Scope4/1
  [V_a] -> Bus Creator/10  "Va"

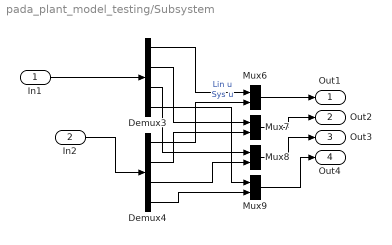
== system pada_plant_model_testing/Subsystem ==
  In1 : Inport
  In2 : Inport  Port=2
  Demux3 : Demux
  Demux4 : Demux
  Mux{6..9} (4 alike) : Mux  Inputs=2
  Out1 : Outport
  Out2 : Outport  Port=2
  Out3 : Outport  Port=3
  Out4 : Outport  Port=4
  wires:
  Demux4/4 -> Mux9/2
  Demux3/2 -> Mux7/1
  Demux4/1 -> Mux6/2  "Sys u"
  Demux4/2 -> Mux7/2
  Demux4/3 -> Mux8/2
  In2/1 -> Demux4/1
  Demux3/4 -> Mux9/1
  Demux3/1 -> Mux6/1  "Lin u"
  Demux3/3 -> Mux8/1
  Mux6/1 -> Out1/1
  Mux8/1 -> Out3/1
  Mux7/1 -> Out2/1
  Mux9/1 -> Out4/1
  In1/1 -> Demux3/1

== system pada_plant_model_testing/Plant1/Aerodynamics ==
  Ele : Inport
  Ail : Inport  Port=2
  AoA : Inport  Port=3
  SSA : Inport  Port=4
  Va : Inport  Port=5
  Aero Coefficients : Subsystem
  Forces and Moments : Subsystem
  F_aero : Outport
  M_aero : Outport  Port=2
  wires:
  AoA/1 -> Forces and Moments/2(AoA), Aero Coefficients/1(AoA)
  Ail/1 -> Aero Coefficients/4(Ail)
  Forces and Moments/2(M_aero) -> M_aero/1
  Ele/1 -> Aero Coefficients/3(Ele)
  Aero Coefficients/1(Coef_stab) -> Forces and Moments/1(Coef_stab)
  Forces and Moments/1(F_aero) -> F_aero/1
  SSA/1 -> Aero Coefficients/2(SSA)
  Va/1 -> Forces and Moments/3(Va)

== system pada_plant_model_testing/Plant1/Gravity ==
  Pitch : Inport
  Roll : Inport  Port=2
  Constant : Constant  Value=m
  Constant1 : Constant  Value=g
  MATLAB Function1 : MATLAB Function  TreatAsAtomicUnit=on
  F_grav : Outport
  wires:
  Pitch/1 -> MATLAB Function1/1(pitch)
  MATLAB Function1/1(F_grav) -> F_grav/1
  Constant/1 -> MATLAB Function1/3(m)
  Constant1/1 -> MATLAB Function1/4(g)
  Roll/1 -> MATLAB Function1/2(roll)

== system pada_plant_model_testing/Plant1/Propulsion ==
  Thr : Inport
  Va : Inport  Port=2
  Constant : Constant  Value=S_prop
  Constant1 : Constant  Value=k_motor
  Constant2 : Constant  Value=rho
  MATLAB Function1 : MATLAB Function  TreatAsAtomicUnit=on
  F_prop : Outport
  wires:
  MATLAB Function1/1(F_prop) -> F_prop/1
  Va/1 -> MATLAB Function1/2(Va)
  Constant2/1 -> MATLAB Function1/3(rho)
  Constant1/1 -> MATLAB Function1/5(k_motor)
  Constant/1 -> MATLAB Function1/4(S_prop)
  Thr/1 -> MATLAB Function1/1(Thr)

== system pada_plant_model_testing/Plant1/States ==
  States : Inport
  Bus Selector : BusSelector  OutputSignals=Vb,att,d_att
  Demux : Demux  Outputs=3
  Demux2 : Demux  Outputs=3
  Demux4 : Demux  Outputs=3
  Mux : Mux
  Mux2 : Mux  Inputs=5
  Lon_States : Outport
  Lat_States : Outport  Port=2
  wires:
  Demux/1 -> Mux/1  "u"
  Bus Selector/3 -> Demux4/1  "<d_att>"
  Demux/3 -> Mux/2  "w"
  Bus Selector/2 -> Demux2/1  "<att>"
  Demux4/2 -> Mux/3  "q"
  Demux2/1 -> Mux2/4  "phi"
  Bus Selector/1 -> Demux/1  "<Vb>"
  States/1 -> Bus Selector/1
  Demux/2 -> Mux2/1  "v"
  Demux4/3 -> Mux2/3  "r"
  Demux2/2 -> Mux/4  "theta"
  Demux4/1 -> Mux2/2  "p"
  Mux/1 -> Lon_States/1
  Mux2/1 -> Lat_States/1
  Demux2/3 -> Mux2/5  "psi"

== system pada_plant_model_testing/Plant2/Aerodynamics ==
  Ele : Inport
  Ail : Inport  Port=2
  AoA : Inport  Port=3
  SSA : Inport  Port=4
  Va : Inport  Port=5
  Aero Coefficients : Subsystem
  Forces and Moments : Subsystem
  F_aero : Outport
  M_aero : Outport  Port=2
  wires:
  AoA/1 -> Forces and Moments/2(AoA), Aero Coefficients/1(AoA)
  Ail/1 -> Aero Coefficients/4(Ail)
  Forces and Moments/2(M_aero) -> M_aero/1
  Ele/1 -> Aero Coefficients/3(Ele)
  Aero Coefficients/1(Coef_stab) -> Forces and Moments/1(Coef_stab)
  Forces and Moments/1(F_aero) -> F_aero/1
  SSA/1 -> Aero Coefficients/2(SSA)
  Va/1 -> Forces and Moments/3(Va)

== system pada_plant_model_testing/Plant2/Gravity ==
  Pitch : Inport
  Roll : Inport  Port=2
  Constant : Constant  Value=m
  Constant1 : Constant  Value=g
  MATLAB Function1 : MATLAB Function  TreatAsAtomicUnit=on
  F_grav : Outport
  wires:
  Pitch/1 -> MATLAB Function1/1(pitch)
  MATLAB Function1/1(F_grav) -> F_grav/1
  Constant/1 -> MATLAB Function1/3(m)
  Constant1/1 -> MATLAB Function1/4(g)
  Roll/1 -> MATLAB Function1/2(roll)

== system pada_plant_model_testing/Plant2/Propulsion ==
  Thr : Inport
  Va : Inport  Port=2
  Constant : Constant  Value=S_prop
  Constant1 : Constant  Value=k_motor
  Constant2 : Constant  Value=rho
  MATLAB Function1 : MATLAB Function  TreatAsAtomicUnit=on
  F_prop : Outport
  wires:
  MATLAB Function1/1(F_prop) -> F_prop/1
  Va/1 -> MATLAB Function1/2(Va)
  Constant2/1 -> MATLAB Function1/3(rho)
  Constant1/1 -> MATLAB Function1/5(k_motor)
  Constant/1 -> MATLAB Function1/4(S_prop)
  Thr/1 -> MATLAB Function1/1(Thr)

== system pada_plant_model_testing/Plant2/States ==
  States : Inport
  Bus Selector : BusSelector  OutputSignals=Vb,att,d_att
  Demux : Demux  Outputs=3
  Demux2 : Demux  Outputs=3
  Demux4 : Demux  Outputs=3
  Mux : Mux
  Mux2 : Mux  Inputs=5
  Lon_States : Outport
  Lat_States : Outport  Port=2
  wires:
  Demux/1 -> Mux/1  "u"
  Bus Selector/3 -> Demux4/1  "<d_att>"
  Demux/3 -> Mux/2  "w"
  Bus Selector/2 -> Demux2/1  "<att>"
  Demux4/2 -> Mux/3  "q"
  Demux2/1 -> Mux2/4  "phi"
  Bus Selector/1 -> Demux/1  "<Vb>"
  States/1 -> Bus Selector/1
  Demux/2 -> Mux2/1  "v"
  Demux4/3 -> Mux2/3  "r"
  Demux2/2 -> Mux/4  "theta"
  Demux4/1 -> Mux2/2  "p"
  Mux/1 -> Lon_States/1
  Mux2/1 -> Lat_States/1
  Demux2/3 -> Mux2/5  "psi"

== system pada_plant_model_testing/Plant3/Aerodynamics ==
  Ele : Inport
  Ail : Inport  Port=2
  AoA : Inport  Port=3
  SSA : Inport  Port=4
  Va : Inport  Port=5
  Aero Coefficients : Subsystem
  Forces and Moments : Subsystem
  F_aero : Outport
  M_aero : Outport  Port=2
  wires:
  AoA/1 -> Forces and Moments/2(AoA), Aero Coefficients/1(AoA)
  Ail/1 -> Aero Coefficients/4(Ail)
  Forces and Moments/2(M_aero) -> M_aero/1
  Ele/1 -> Aero Coefficients/3(Ele)
  Aero Coefficients/1(Coef_stab) -> Forces and Moments/1(Coef_stab)
  Forces and Moments/1(F_aero) -> F_aero/1
  SSA/1 -> Aero Coefficients/2(SSA)
  Va/1 -> Forces and Moments/3(Va)

== system pada_plant_model_testing/Plant3/Gravity ==
  Pitch : Inport
  Roll : Inport  Port=2
  Constant : Constant  Value=m
  Constant1 : Constant  Value=g
  MATLAB Function1 : MATLAB Function  TreatAsAtomicUnit=on
  F_grav : Outport
  wires:
  Pitch/1 -> MATLAB Function1/1(pitch)
  MATLAB Function1/1(F_grav) -> F_grav/1
  Constant/1 -> MATLAB Function1/3(m)
  Constant1/1 -> MATLAB Function1/4(g)
  Roll/1 -> MATLAB Function1/2(roll)

== system pada_plant_model_testing/Plant3/Propulsion ==
  Thr : Inport
  Va : Inport  Port=2
  Constant : Constant  Value=S_prop
  Constant1 : Constant  Value=k_motor
  Constant2 : Constant  Value=rho
  MATLAB Function1 : MATLAB Function  TreatAsAtomicUnit=on
  F_prop : Outport
  wires:
  MATLAB Function1/1(F_prop) -> F_prop/1
  Va/1 -> MATLAB Function1/2(Va)
  Constant2/1 -> MATLAB Function1/3(rho)
  Constant1/1 -> MATLAB Function1/5(k_motor)
  Constant/1 -> MATLAB Function1/4(S_prop)
  Thr/1 -> MATLAB Function1/1(Thr)

== system pada_plant_model_testing/Plant3/States ==
  States : Inport
  Bus Selector : BusSelector  OutputSignals=Vb,att,d_att
  Demux : Demux  Outputs=3
  Demux2 : Demux  Outputs=3
  Demux4 : Demux  Outputs=3
  Mux : Mux
  Mux2 : Mux  Inputs=5
  Lon_States : Outport
  Lat_States : Outport  Port=2
  wires:
  Demux/1 -> Mux/1  "u"
  Bus Selector/3 -> Demux4/1  "<d_att>"
  Demux/3 -> Mux/2  "w"
  Bus Selector/2 -> Demux2/1  "<att>"
  Demux4/2 -> Mux/3  "q"
  Demux2/1 -> Mux2/4  "phi"
  Bus Selector/1 -> Demux/1  "<Vb>"
  States/1 -> Bus Selector/1
  Demux/2 -> Mux2/1  "v"
  Demux4/3 -> Mux2/3  "r"
  Demux2/2 -> Mux/4  "theta"
  Demux4/1 -> Mux2/2  "p"
  Mux/1 -> Lon_States/1
  Mux2/1 -> Lat_States/1
  Demux2/3 -> Mux2/5  "psi"

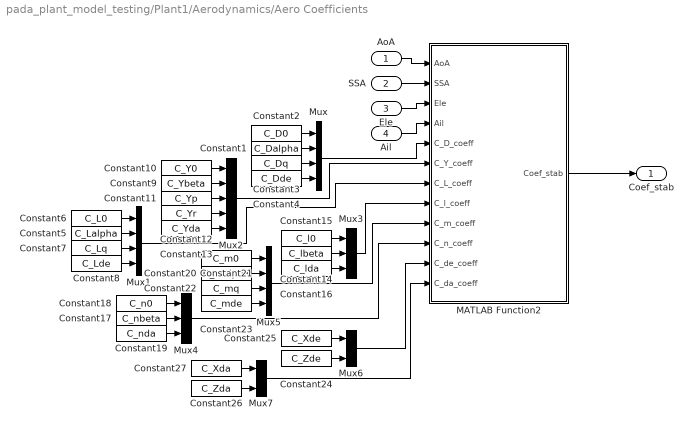
== system pada_plant_model_testing/Plant1/Aerodynamics/Aero Coefficients ==
  AoA : Inport
  SSA : Inport  Port=2
  Ele : Inport  Port=3
  Ail : Inport  Port=4
  Constant1 : Constant  Value=C_Dalpha
  Constant10 : Constant  Value=C_Y0
  Constant11 : Constant  Value=C_Yp
  Constant12 : Constant  Value=C_Yr
  Constant13 : Constant  Value=C_Yda
  Constant14 : Constant  Value=C_lbeta
  Constant15 : Constant  Value=C_l0
  Constant16 : Constant  Value=C_lda
  Constant17 : Constant  Value=C_nbeta
  Constant18 : Constant  Value=C_n0
  Constant19 : Constant  Value=C_nda
  Constant2 : Constant  Value=C_D0
  Constant20 : Constant  Value=C_malpha
  Constant21 : Constant  Value=C_m0
  Constant22 : Constant  Value=C_mq
  Constant23 : Constant  Value=C_mde
  Constant24 : Constant  Value=C_Zde
  Constant25 : Constant  Value=C_Xde
  Constant26 : Constant  Value=C_Zda
  Constant27 : Constant  Value=C_Xda
  Constant3 : Constant  Value=C_Dq
  Constant4 : Constant  Value=C_Dde
  Constant5 : Constant  Value=C_Lalpha
  Constant6 : Constant  Value=C_L0
  Constant7 : Constant  Value=C_Lq
  Constant8 : Constant  Value=C_Lde
  Constant9 : Constant  Value=C_Ybeta
  MATLAB Function2 : MATLAB Function  TreatAsAtomicUnit=on
  Mux : Mux
  Mux1 : Mux
  Mux2 : Mux  Inputs=5
  Mux3 : Mux  Inputs=3
  Mux4 : Mux  Inputs=3
  Mux5 : Mux
  Mux6 : Mux  Inputs=2
  Mux7 : Mux  Inputs=2
  Coef_stab : Outport
  wires:
  Constant23/1 -> Mux5/4
  Mux3/1 -> MATLAB Function2/8(C_l_coeff)
  Constant17/1 -> Mux4/2
  Constant14/1 -> Mux3/2
  Constant4/1 -> Mux/4
  Constant12/1 -> Mux2/4
  Mux2/1 -> MATLAB Function2/6(C_Y_coeff)
  Constant19/1 -> Mux4/3
  Constant18/1 -> Mux4/1
  Mux4/1 -> MATLAB Function2/10(C_n_coeff)
  Mux5/1 -> MATLAB Function2/9(C_m_coeff)
  Constant15/1 -> Mux3/1
  Constant16/1 -> Mux3/3
  SSA/1 -> MATLAB Function2/2(SSA)
  Constant7/1 -> Mux1/3
  Constant20/1 -> Mux5/2
  Constant5/1 -> Mux1/2
  Constant6/1 -> Mux1/1
  Constant8/1 -> Mux1/4
  Constant2/1 -> Mux/1
  MATLAB Function2/1(Coef_stab) -> Coef_stab/1
  Constant22/1 -> Mux5/3
  Constant9/1 -> Mux2/2
  Constant11/1 -> Mux2/3
  AoA/1 -> MATLAB Function2/1(AoA)
  Constant10/1 -> Mux2/1
  Mux/1 -> MATLAB Function2/5(C_D_coeff)
  Constant21/1 -> Mux5/1
  Constant3/1 -> Mux/3
  Constant13/1 -> Mux2/5
  Mux1/1 -> MATLAB Function2/7(C_L_coeff)
  Constant1/1 -> Mux/2
  Ele/1 -> MATLAB Function2/3(Ele)
  Ail/1 -> MATLAB Function2/4(Ail)
  Constant25/1 -> Mux6/1
  Constant24/1 -> Mux6/2
  Constant27/1 -> Mux7/1
  Constant26/1 -> Mux7/2
  Mux6/1 -> MATLAB Function2/11(C_de_coeff)
  Mux7/1 -> MATLAB Function2/12(C_da_coeff)

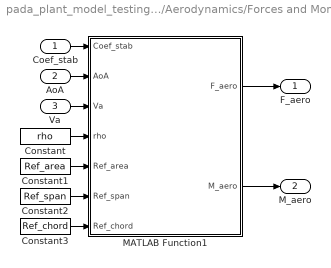
== system pada_plant_model_testing/Plant1/Aerodynamics/Forces and Moments ==
  Coef_stab : Inport
  AoA : Inport  Port=2
  Va : Inport  Port=3
  Constant : Constant  Value=rho
  Constant1 : Constant  Value=Ref_area
  Constant2 : Constant  Value=Ref_span
  Constant3 : Constant  Value=Ref_chord
  MATLAB Function1 : MATLAB Function  TreatAsAtomicUnit=on
  F_aero : Outport
  M_aero : Outport  Port=2
  wires:
  Constant3/1 -> MATLAB Function1/7(Ref_chord)
  Va/1 -> MATLAB Function1/3(Va)
  Constant1/1 -> MATLAB Function1/5(Ref_area)
  Constant/1 -> MATLAB Function1/4(rho)
  Coef_stab/1 -> MATLAB Function1/1(Coef_stab)
  AoA/1 -> MATLAB Function1/2(AoA)
  Constant2/1 -> MATLAB Function1/6(Ref_span)
  MATLAB Function1/1(F_aero) -> F_aero/1
  MATLAB Function1/2(M_aero) -> M_aero/1

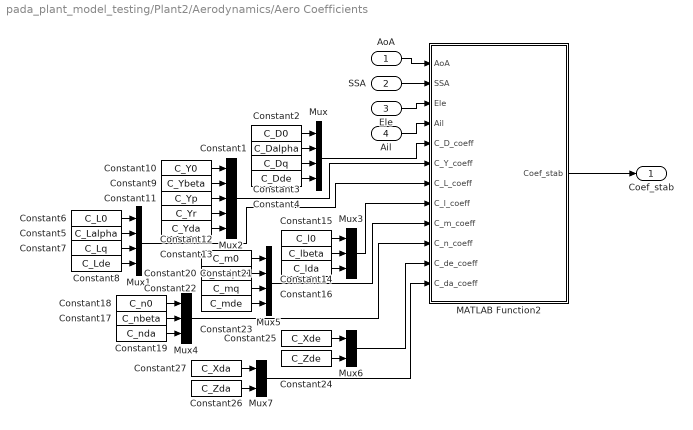
== system pada_plant_model_testing/Plant2/Aerodynamics/Aero Coefficients ==
  AoA : Inport
  SSA : Inport  Port=2
  Ele : Inport  Port=3
  Ail : Inport  Port=4
  Constant1 : Constant  Value=C_Dalpha
  Constant10 : Constant  Value=C_Y0
  Constant11 : Constant  Value=C_Yp
  Constant12 : Constant  Value=C_Yr
  Constant13 : Constant  Value=C_Yda
  Constant14 : Constant  Value=C_lbeta
  Constant15 : Constant  Value=C_l0
  Constant16 : Constant  Value=C_lda
  Constant17 : Constant  Value=C_nbeta
  Constant18 : Constant  Value=C_n0
  Constant19 : Constant  Value=C_nda
  Constant2 : Constant  Value=C_D0
  Constant20 : Constant  Value=C_malpha
  Constant21 : Constant  Value=C_m0
  Constant22 : Constant  Value=C_mq
  Constant23 : Constant  Value=C_mde
  Constant24 : Constant  Value=C_Zde
  Constant25 : Constant  Value=C_Xde
  Constant26 : Constant  Value=C_Zda
  Constant27 : Constant  Value=C_Xda
  Constant3 : Constant  Value=C_Dq
  Constant4 : Constant  Value=C_Dde
  Constant5 : Constant  Value=C_Lalpha
  Constant6 : Constant  Value=C_L0
  Constant7 : Constant  Value=C_Lq
  Constant8 : Constant  Value=C_Lde
  Constant9 : Constant  Value=C_Ybeta
  MATLAB Function2 : MATLAB Function  TreatAsAtomicUnit=on
  Mux : Mux
  Mux1 : Mux
  Mux2 : Mux  Inputs=5
  Mux3 : Mux  Inputs=3
  Mux4 : Mux  Inputs=3
  Mux5 : Mux
  Mux6 : Mux  Inputs=2
  Mux7 : Mux  Inputs=2
  Coef_stab : Outport
  wires:
  Constant23/1 -> Mux5/4
  Mux3/1 -> MATLAB Function2/8(C_l_coeff)
  Constant17/1 -> Mux4/2
  Constant14/1 -> Mux3/2
  Constant4/1 -> Mux/4
  Constant12/1 -> Mux2/4
  Mux2/1 -> MATLAB Function2/6(C_Y_coeff)
  Constant19/1 -> Mux4/3
  Constant18/1 -> Mux4/1
  Mux4/1 -> MATLAB Function2/10(C_n_coeff)
  Mux5/1 -> MATLAB Function2/9(C_m_coeff)
  Constant15/1 -> Mux3/1
  Constant16/1 -> Mux3/3
  SSA/1 -> MATLAB Function2/2(SSA)
  Constant7/1 -> Mux1/3
  Constant20/1 -> Mux5/2
  Constant5/1 -> Mux1/2
  Constant6/1 -> Mux1/1
  Constant8/1 -> Mux1/4
  Constant2/1 -> Mux/1
  MATLAB Function2/1(Coef_stab) -> Coef_stab/1
  Constant22/1 -> Mux5/3
  Constant9/1 -> Mux2/2
  Constant11/1 -> Mux2/3
  AoA/1 -> MATLAB Function2/1(AoA)
  Constant10/1 -> Mux2/1
  Mux/1 -> MATLAB Function2/5(C_D_coeff)
  Constant21/1 -> Mux5/1
  Constant3/1 -> Mux/3
  Constant13/1 -> Mux2/5
  Mux1/1 -> MATLAB Function2/7(C_L_coeff)
  Constant1/1 -> Mux/2
  Ele/1 -> MATLAB Function2/3(Ele)
  Ail/1 -> MATLAB Function2/4(Ail)
  Constant25/1 -> Mux6/1
  Constant24/1 -> Mux6/2
  Constant27/1 -> Mux7/1
  Constant26/1 -> Mux7/2
  Mux6/1 -> MATLAB Function2/11(C_de_coeff)
  Mux7/1 -> MATLAB Function2/12(C_da_coeff)

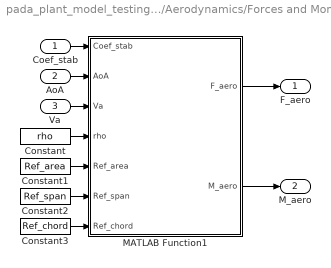
== system pada_plant_model_testing/Plant2/Aerodynamics/Forces and Moments ==
  Coef_stab : Inport
  AoA : Inport  Port=2
  Va : Inport  Port=3
  Constant : Constant  Value=rho
  Constant1 : Constant  Value=Ref_area
  Constant2 : Constant  Value=Ref_span
  Constant3 : Constant  Value=Ref_chord
  MATLAB Function1 : MATLAB Function  TreatAsAtomicUnit=on
  F_aero : Outport
  M_aero : Outport  Port=2
  wires:
  Constant3/1 -> MATLAB Function1/7(Ref_chord)
  Va/1 -> MATLAB Function1/3(Va)
  Constant1/1 -> MATLAB Function1/5(Ref_area)
  Constant/1 -> MATLAB Function1/4(rho)
  Coef_stab/1 -> MATLAB Function1/1(Coef_stab)
  AoA/1 -> MATLAB Function1/2(AoA)
  Constant2/1 -> MATLAB Function1/6(Ref_span)
  MATLAB Function1/1(F_aero) -> F_aero/1
  MATLAB Function1/2(M_aero) -> M_aero/1

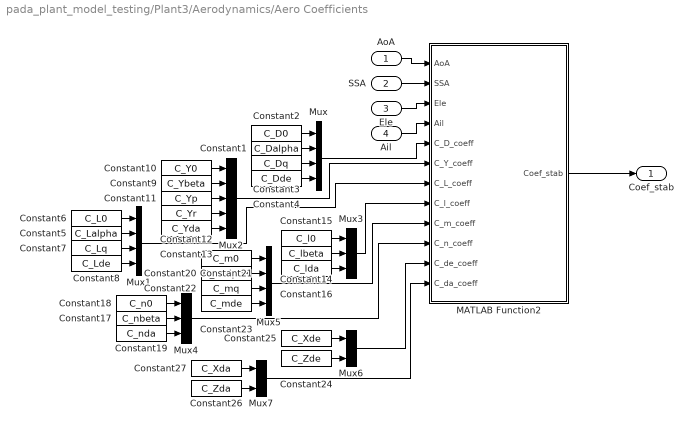
== system pada_plant_model_testing/Plant3/Aerodynamics/Aero Coefficients ==
  AoA : Inport
  SSA : Inport  Port=2
  Ele : Inport  Port=3
  Ail : Inport  Port=4
  Constant1 : Constant  Value=C_Dalpha
  Constant10 : Constant  Value=C_Y0
  Constant11 : Constant  Value=C_Yp
  Constant12 : Constant  Value=C_Yr
  Constant13 : Constant  Value=C_Yda
  Constant14 : Constant  Value=C_lbeta
  Constant15 : Constant  Value=C_l0
  Constant16 : Constant  Value=C_lda
  Constant17 : Constant  Value=C_nbeta
  Constant18 : Constant  Value=C_n0
  Constant19 : Constant  Value=C_nda
  Constant2 : Constant  Value=C_D0
  Constant20 : Constant  Value=C_malpha
  Constant21 : Constant  Value=C_m0
  Constant22 : Constant  Value=C_mq
  Constant23 : Constant  Value=C_mde
  Constant24 : Constant  Value=C_Zde
  Constant25 : Constant  Value=C_Xde
  Constant26 : Constant  Value=C_Zda
  Constant27 : Constant  Value=C_Xda
  Constant3 : Constant  Value=C_Dq
  Constant4 : Constant  Value=C_Dde
  Constant5 : Constant  Value=C_Lalpha
  Constant6 : Constant  Value=C_L0
  Constant7 : Constant  Value=C_Lq
  Constant8 : Constant  Value=C_Lde
  Constant9 : Constant  Value=C_Ybeta
  MATLAB Function2 : MATLAB Function  TreatAsAtomicUnit=on
  Mux : Mux
  Mux1 : Mux
  Mux2 : Mux  Inputs=5
  Mux3 : Mux  Inputs=3
  Mux4 : Mux  Inputs=3
  Mux5 : Mux
  Mux6 : Mux  Inputs=2
  Mux7 : Mux  Inputs=2
  Coef_stab : Outport
  wires:
  Constant23/1 -> Mux5/4
  Mux3/1 -> MATLAB Function2/8(C_l_coeff)
  Constant17/1 -> Mux4/2
  Constant14/1 -> Mux3/2
  Constant4/1 -> Mux/4
  Constant12/1 -> Mux2/4
  Mux2/1 -> MATLAB Function2/6(C_Y_coeff)
  Constant19/1 -> Mux4/3
  Constant18/1 -> Mux4/1
  Mux4/1 -> MATLAB Function2/10(C_n_coeff)
  Mux5/1 -> MATLAB Function2/9(C_m_coeff)
  Constant15/1 -> Mux3/1
  Constant16/1 -> Mux3/3
  SSA/1 -> MATLAB Function2/2(SSA)
  Constant7/1 -> Mux1/3
  Constant20/1 -> Mux5/2
  Constant5/1 -> Mux1/2
  Constant6/1 -> Mux1/1
  Constant8/1 -> Mux1/4
  Constant2/1 -> Mux/1
  MATLAB Function2/1(Coef_stab) -> Coef_stab/1
  Constant22/1 -> Mux5/3
  Constant9/1 -> Mux2/2
  Constant11/1 -> Mux2/3
  AoA/1 -> MATLAB Function2/1(AoA)
  Constant10/1 -> Mux2/1
  Mux/1 -> MATLAB Function2/5(C_D_coeff)
  Constant21/1 -> Mux5/1
  Constant3/1 -> Mux/3
  Constant13/1 -> Mux2/5
  Mux1/1 -> MATLAB Function2/7(C_L_coeff)
  Constant1/1 -> Mux/2
  Ele/1 -> MATLAB Function2/3(Ele)
  Ail/1 -> MATLAB Function2/4(Ail)
  Constant25/1 -> Mux6/1
  Constant24/1 -> Mux6/2
  Constant27/1 -> Mux7/1
  Constant26/1 -> Mux7/2
  Mux6/1 -> MATLAB Function2/11(C_de_coeff)
  Mux7/1 -> MATLAB Function2/12(C_da_coeff)
